simulink model "imuTester"  (R2024b)
settings: Solver=FixedStepAuto  StartTime=0.0  StopTime=8000  FixedStep=1/imuHz  RelTol=1e-3
InitFcn:
  | accelParamFile = './Resources/Calibrations/accel_accel0_20251211_allan_stable.mat';
  | gyroParamFile = './Resources/Calibrations/gyro_gyro0_20251211_allan.mat';
  | 
  | accelCalib = load(accelParamFile);
  | gyroCalib = load(gyroParamFile);
  | 
  | imuHz = 8000;
undefined symbols (not defined in the file or in its folder): fractalcoef
libraries: mspsensorlib x4
settings Model: Creator=Alyssa  LastModifiedBy=Alyssa

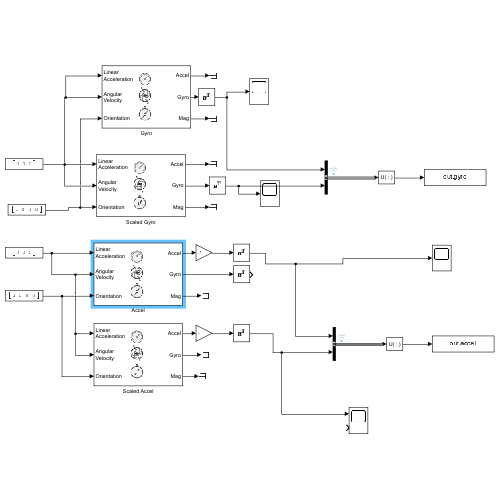
[thumbnail: Simulink's stored preview of the top-level diagram]
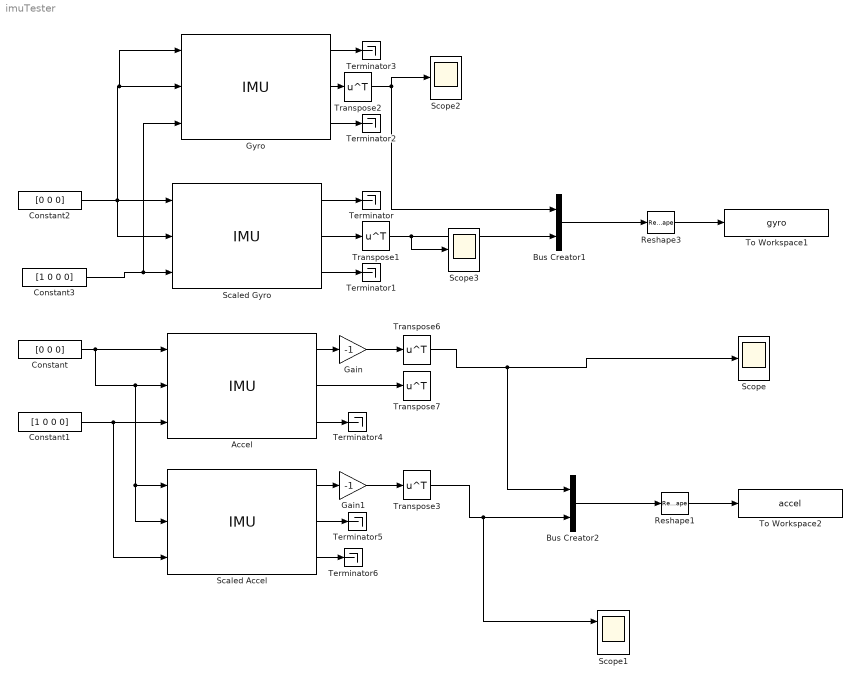
== system imuTester ==
  Accel : mspsensorlib/IMU  DispRefFrame=NED  TemperaturePort=off  Temperature=25  MagneticFieldPort=off  MagneticFieldNED=[25.015, -4.798, -22.615];%[ 27.5550, -2.4169, -16.0849 ]  MagneticFieldENU=[ -2.4169, 27.5550, 16.0849 ]  SeedDouble=67  SimulateUsing=Interpreted execution  AccelParamsMeasurementRange=accelCalib.max  AccelParamsResolution=accelCalib.res  AccelParamsConstantBias=accelCalib.simBias  AccelParamsAxesMisalignment=accelCalib.skew  AccelParamsNoiseDensity=accelCalib.vrw%*0.6  AccelParamsBiasInstability=accelCalib.bi  AccelParamsBiasInstabilityNumerator=fractalcoef().Numerator  AccelParamsBiasInstabilityDenominator=fractalcoef().Denominator  AccelParamsRandomWalk=accelCalib.rrw  AccelParamsNoiseType=single-sided  AccelParamsTemperatureBias=[ 0, 0, 0 ]  AccelParamsTemperatureScaleFactor=[ 0, 0, 0 ]  GyroParamsMeasurementRange=gyroCalib.max  GyroParamsResolution=gyroCalib.res  GyroParamsConstantBias=gyroCalib.simBias  GyroParamsAxesMisalignment=gyroCalib.skew  GyroParamsAccelerationBias=[ 0, 0, 0 ]  GyroParamsNoiseDensity=gyroCalib.arw  GyroParamsBiasInstability=gyroCalib.bi  GyroParamsBiasInstabilityNumerator=fractalcoef().Numerator  GyroParamsBiasInstabilityDenominator=fractalcoef().Denominator  GyroParamsRandomWalk=gyroCalib.rrw  GyroParamsNoiseType=single-sided  GyroParamsTemperatureBias=[ 0, 0, 0 ]  GyroParamsTemperatureScaleFactor=[ 0, 0, 0 ]  MagParamsMeasurementRange=Inf  MagParamsResolution=0  MagParamsConstantBias=[ 0, 0, 0 ]  MagParamsAxesMisalignment=[ 100, 0, 0; 0, 100, 0; 0, 0, 100 ]  MagParamsNoiseDensity=[ 0, 0, 0 ]  MagParamsBiasInstability=[ 0, 0, 0 ]  MagParamsBiasInstabilityNumerator=fractalcoef().Numerator  MagParamsBiasInstabilityDenominator=fractalcoef().Denominator  MagParamsRandomWalk=[ 0, 0, 0 ]  MagParamsNoiseType=double-sided  MagParamsTemperatureBias=[ 0, 0, 0 ]  MagParamsTemperatureScaleFactor=[ 0, 0, 0 ]
  Bus Creator1 : BusCreator  Inputs=2
  Bus Creator2 : BusCreator  Inputs=2
  Constant : Constant  Value=[0 0 0]  VectorParams1D=off
  Constant1 : Constant  Value=[1 0 0 0]  VectorParams1D=off
  Constant2 : Constant  Value=[0 0 0]  VectorParams1D=off  SampleTime=1/2000
  Constant3 : Constant  Value=[1 0 0 0]  VectorParams1D=off  SampleTime=1/2000
  Gain : Gain  Gain=-1
  Gain1 : Gain  Gain=-1
  Gyro : mspsensorlib/IMU  DispRefFrame=NED  TemperaturePort=off  Temperature=25  MagneticFieldPort=off  MagneticFieldNED=[25.015, -4.798, -22.615];%[ 27.5550, -2.4169, -16.0849 ]  MagneticFieldENU=[ -2.4169, 27.5550, 16.0849 ]  SeedDouble=67  SimulateUsing=Interpreted execution  AccelParamsMeasurementRange=accelCalib.max  AccelParamsResolution=accelCalib.res  AccelParamsConstantBias=accelCalib.simBias  AccelParamsAxesMisalignment=accelCalib.skew  AccelParamsNoiseDensity=accelCalib.vrw%*0.6  AccelParamsBiasInstability=accelCalib.bi  AccelParamsBiasInstabilityNumerator=fractalcoef().Numerator  AccelParamsBiasInstabilityDenominator=fractalcoef().Denominator  AccelParamsRandomWalk=accelCalib.rrw  AccelParamsNoiseType=single-sided  AccelParamsTemperatureBias=[ 0, 0, 0 ]  AccelParamsTemperatureScaleFactor=[ 0, 0, 0 ]  GyroParamsMeasurementRange=gyroCalib.max  GyroParamsResolution=gyroCalib.res  GyroParamsConstantBias=gyroCalib.simBias  GyroParamsAxesMisalignment=gyroCalib.skew  GyroParamsAccelerationBias=[ 0, 0, 0 ]  GyroParamsNoiseDensity=gyroCalib.arw%*2  GyroParamsBiasInstability=gyroCalib.bi  GyroParamsBiasInstabilityNumerator=fractalcoef().Numerator  GyroParamsBiasInstabilityDenominator=fractalcoef().Denominator  GyroParamsRandomWalk=gyroCalib.rrw  GyroParamsNoiseType=single-sided  GyroParamsTemperatureBias=[ 0, 0, 0 ]  GyroParamsTemperatureScaleFactor=[ 0, 0, 0 ]  MagParamsMeasurementRange=Inf  MagParamsResolution=0  MagParamsConstantBias=[ 0, 0, 0 ]  MagParamsAxesMisalignment=[ 100, 0, 0; 0, 100, 0; 0, 0, 100 ]  MagParamsNoiseDensity=[ 0, 0, 0 ]  MagParamsBiasInstability=[ 0, 0, 0 ]  MagParamsBiasInstabilityNumerator=fractalcoef().Numerator  MagParamsBiasInstabilityDenominator=fractalcoef().Denominator  MagParamsRandomWalk=[ 0, 0, 0 ]  MagParamsNoiseType=double-sided  MagParamsTemperatureBias=[ 0, 0, 0 ]  MagParamsTemperatureScaleFactor=[ 0, 0, 0 ]
  Reshape1 : Reshape
  Reshape3 : Reshape
  Scaled Accel : mspsensorlib/IMU  DispRefFrame=NED  TemperaturePort=off  Temperature=25  MagneticFieldPort=off  MagneticFieldNED=[25.015, -4.798, -22.615];%[ 27.5550, -2.4169, -16.0849 ]  MagneticFieldENU=[ -2.4169, 27.5550, 16.0849 ]  SeedDouble=67  SimulateUsing=Interpreted execution  AccelParamsMeasurementRange=accelCalib.max  AccelParamsResolution=accelCalib.res  AccelParamsConstantBias=accelCalib.simBias  AccelParamsAxesMisalignment=accelCalib.skew  AccelParamsNoiseDensity=accelCalib.vrw*0.6  AccelParamsBiasInstability=accelCalib.bi  AccelParamsBiasInstabilityNumerator=fractalcoef().Numerator  AccelParamsBiasInstabilityDenominator=fractalcoef().Denominator  AccelParamsRandomWalk=accelCalib.rrw  AccelParamsNoiseType=single-sided  AccelParamsTemperatureBias=[ 0, 0, 0 ]  AccelParamsTemperatureScaleFactor=[ 0, 0, 0 ]  GyroParamsMeasurementRange=gyroCalib.max  GyroParamsResolution=gyroCalib.res  GyroParamsConstantBias=gyroCalib.simBias  GyroParamsAxesMisalignment=gyroCalib.skew  GyroParamsAccelerationBias=[ 0, 0, 0 ]  GyroParamsNoiseDensity=gyroCalib.arw  GyroParamsBiasInstability=gyroCalib.bi  GyroParamsBiasInstabilityNumerator=fractalcoef().Numerator  GyroParamsBiasInstabilityDenominator=fractalcoef().Denominator  GyroParamsRandomWalk=gyroCalib.rrw  GyroParamsNoiseType=single-sided  GyroParamsTemperatureBias=[ 0, 0, 0 ]  GyroParamsTemperatureScaleFactor=[ 0, 0, 0 ]  MagParamsMeasurementRange=Inf  MagParamsResolution=0  MagParamsConstantBias=[ 0, 0, 0 ]  MagParamsAxesMisalignment=[ 100, 0, 0; 0, 100, 0; 0, 0, 100 ]  MagParamsNoiseDensity=[ 0, 0, 0 ]  MagParamsBiasInstability=[ 0, 0, 0 ]  MagParamsBiasInstabilityNumerator=fractalcoef().Numerator  MagParamsBiasInstabilityDenominator=fractalcoef().Denominator  MagParamsRandomWalk=[ 0, 0, 0 ]  MagParamsNoiseType=double-sided  MagParamsTemperatureBias=[ 0, 0, 0 ]  MagParamsTemperatureScaleFactor=[ 0, 0, 0 ]
  Scaled Gyro : mspsensorlib/IMU  DispRefFrame=NED  TemperaturePort=off  Temperature=25  MagneticFieldPort=off  MagneticFieldNED=[25.015, -4.798, -22.615];%[ 27.5550, -2.4169, -16.0849 ]  MagneticFieldENU=[ -2.4169, 27.5550, 16.0849 ]  SeedDouble=67  SimulateUsing=Interpreted execution  AccelParamsMeasurementRange=accelCalib.max  AccelParamsResolution=accelCalib.res  AccelParamsConstantBias=accelCalib.simBias  AccelParamsAxesMisalignment=accelCalib.skew  AccelParamsNoiseDensity=accelCalib.vrw%*0.6  AccelParamsBiasInstability=accelCalib.bi  AccelParamsBiasInstabilityNumerator=fractalcoef().Numerator  AccelParamsBiasInstabilityDenominator=fractalcoef().Denominator  AccelParamsRandomWalk=accelCalib.rrw  AccelParamsNoiseType=single-sided  AccelParamsTemperatureBias=[ 0, 0, 0 ]  AccelParamsTemperatureScaleFactor=[ 0, 0, 0 ]  GyroParamsMeasurementRange=gyroCalib.max  GyroParamsResolution=gyroCalib.res  GyroParamsConstantBias=gyroCalib.simBias  GyroParamsAxesMisalignment=gyroCalib.skew  GyroParamsAccelerationBias=[ 0, 0, 0 ]  GyroParamsNoiseDensity=gyroCalib.arw*2  GyroParamsBiasInstability=gyroCalib.bi  GyroParamsBiasInstabilityNumerator=fractalcoef().Numerator  GyroParamsBiasInstabilityDenominator=fractalcoef().Denominator  GyroParamsRandomWalk=gyroCalib.rrw  GyroParamsNoiseType=single-sided  GyroParamsTemperatureBias=[ 0, 0, 0 ]  GyroParamsTemperatureScaleFactor=[ 0, 0, 0 ]  MagParamsMeasurementRange=Inf  MagParamsResolution=0  MagParamsConstantBias=[ 0, 0, 0 ]  MagParamsAxesMisalignment=[ 100, 0, 0; 0, 100, 0; 0, 0, 100 ]  MagParamsNoiseDensity=[ 0, 0, 0 ]  MagParamsBiasInstability=[ 0, 0, 0 ]  MagParamsBiasInstabilityNumerator=fractalcoef().Numerator  MagParamsBiasInstabilityDenominator=fractalcoef().Denominator  MagParamsRandomWalk=[ 0, 0, 0 ]  MagParamsNoiseType=double-sided  MagParamsTemperatureBias=[ 0, 0, 0 ]  MagParamsTemperatureScaleFactor=[ 0, 0, 0 ]
  Scope : Scope
  Scope1 : Scope  NumInputPorts=2
  Scope2 : Scope
  Scope3 : Scope
  Terminator{,1..6} (7 alike) : Terminator
  To Workspace1 : ToWorkspace  VariableName=gyro  SaveFormat=Structure With Time  SampleTime=1/2000
  To Workspace2 : ToWorkspace  VariableName=accel  SaveFormat=Structure With Time  SampleTime=1/imuHz
  Transpose{1..3,6..7} (5 alike) : Math  Operator=transpose
  wires:
  Accel/2 -> Transpose7/1
  Accel/1 -> Gain/1
  Constant/1 -> Accel/1, Scaled Accel/2, Scaled Accel/1, Accel/2
  Gain/1 -> Transpose6/1
  Bus Creator1/1 -> Reshape3/1
  Constant1/1 -> Scaled Accel/3, Accel/3
  Reshape3/1 -> To Workspace1/1
  Constant3/1 -> Gyro/3, Scaled Gyro/3
  Transpose2/1 -> Bus Creator1/1, Scope2/1
  Constant2/1 -> Scaled Gyro/2, Gyro/1, Gyro/2, Scaled Gyro/1
  Scaled Gyro/1 -> Terminator/1
  Scaled Gyro/3 -> Terminator1/1
  Gyro/3 -> Terminator2/1
  Gyro/1 -> Terminator3/1
  Transpose6/1 -> Bus Creator2/1, Scope/1
  Reshape1/1 -> To Workspace2/1
  Bus Creator2/1 -> Reshape1/1
  Transpose3/1 -> Scope1/1, Bus Creator2/2
  Scaled Gyro/2 -> Transpose1/1
  Scaled Accel/1 -> Gain1/1
  Transpose1/1 -> Scope3/1, Bus Creator1/2
  Gyro/2 -> Transpose2/1
  Gain1/1 -> Transpose3/1
  Accel/3 -> Terminator4/1
  Scaled Accel/2 -> Terminator5/1
  Scaled Accel/3 -> Terminator6/1
